simulink model "lucrarea3_2_sim"  (R2020b)
settings: Solver=VariableStepAuto  StartTime=0.0  StopTime=10.0  RelTol=1e-3
values from neighbouring files (symbols this model uses):
  lambda = 0.0001    [lucrarea3_2.m]    (also in lucrarea3_3.m)
  nA = 2    [lucrarea3_2.m]    (also in lucrarea3_3.m)
  nB = 1    [lucrarea3_2.m]    (also in lucrarea3_3.m)
  Orizont = 3    [lucrarea3_2.m]    (also in lucrarea3_3.m)
  P = [G1 0 0;fliplr(G2) 0;fliplr(G3)]    [lucrarea3_2.m]    (also in lucrarea3_3.m; lucrarea4_3.m = [z1; z2])
  PSI = [F1 H1;F2 H2;F3 H3]    [lucrarea3_2.m]    (also in lucrarea3_3.m)
  Q = eye(Orizont)    [lucrarea3_2.m]    (also in lucrarea3_3.m; lucrarea4.m = [1 0;0 1]; lucrarea4_2.m = [1, 0; 0, 1]; lucrarea4_3.m = [1, 0; 0, 1])
  R = zeros(N+Orizont,1);R(21:end)=1    [lucrarea3_2.m]    (also in lucrarea3_3.m; lucrarea4.m = 0.1; lucrarea4_2.m = 0.1; lucrarea4_3.m = 0.1)
settings Model: Creator=student  LastModifiedBy=student

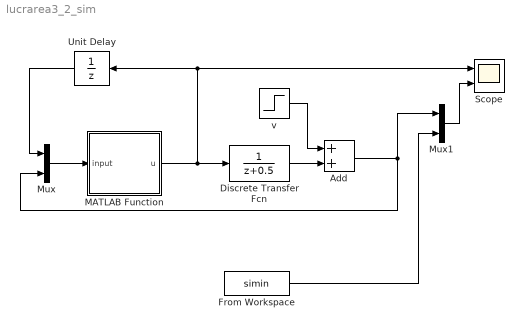
== system lucrarea3_2_sim ==
  Add : Sum
  Discrete Transfer Fcn : DiscreteTransferFcn
  From Workspace : FromWorkspace  VariableName=simin
  MATLAB Function : MATLAB Function  TreatAsAtomicUnit=on
  Mux : Mux  Inputs=2
  Mux1 : Mux  Inputs=2
  Scope : Scope  NumInputPorts=2
  Unit Delay : UnitDelay  SampleTime=-1  HasFrameUpgradeWarning=on
  v : Step  SampleTime=0
  wires:
  Discrete Transfer Fcn/1 -> Add/2
  v/1 -> Add/1
  Mux/1 -> MATLAB Function/1(input)
  MATLAB Function/1(u) -> Scope/1, Unit Delay/1, Discrete Transfer Fcn/1
  Unit Delay/1 -> Mux/1
  Add/1 -> Mux1/1, Mux/2
  From Workspace/1 -> Mux1/2
  Mux1/1 -> Scope/2

== matlab function lucrarea3_2_sim/MATLAB Function ==
  data: input input; u output; R parameter; P parameter; Q parameter; PSI parameter; nA parameter; nB parameter; lambda parameter; Orizont parameter
% ------------------myMPC.m----------------------- %
function u = myMPC(input, R, P, Q, PSI, nA, nB, lambda, Orizont)
% to clear persistent vars in Fcn, call >>clear 'FcnName' in prompt
% clear myMPC
persistent yPast uPast k
if isempty(yPast) % initializari variabile persistente la prima rulare
yPast = zeros(2,1);
uPast = zeros(1,1);
k = 0;
end
% actualizare uPast
for i = length(uPast):-1:2
uPast(i) = uPast(i-1);
end
uPast(1) = input(1);
%%%%%%%%%%%%%%%%%%
% actualizare yPast
for i = length(yPast):-1:2
yPast(i) = yPast(i-1);
end
yPast(1) = input(2);
%%%%%%%%%%%%%%%%%%
Rs = [R(k+1) R(k+1) R(k+1)]';
% eyeO=[1 0 0;0 1 0;0 0 1];
Sol = -inv(P'*Q*P + lambda*eye(3)) * P' * Q * (PSI*[yPast;uPast]-Rs);
u = Sol(1);
k = k+1; %salt la pasul urmator
end % end myMPC
%-----------------------------------------------------------%
